simulink model "SFunctionModel"  (R2023b)
settings: Solver=VariableStepAuto  StartTime=0.0  StopTime=10.0  RelTol=1e-3
libraries: autolibshared x1
settings Model: Creator=Lenovo  LastModifiedBy=Lenovo

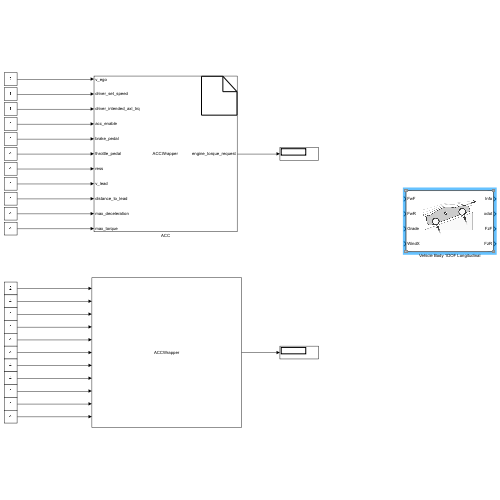
[thumbnail: Simulink's stored preview of the top-level diagram]
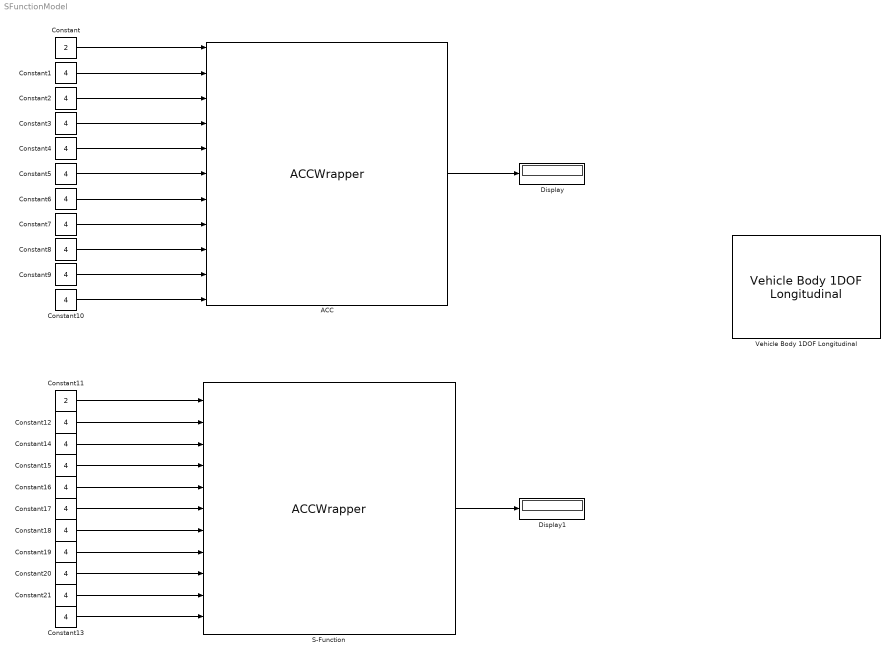
== system SFunctionModel ==
  ACC : S-Function  FunctionName=ACCWrapper  Parameters=1,4,1,1,1,1,1,1,1,1,1  SFunctionModules=ACCWrapper_wrapper.cpp  SFunctionDeploymentMode=off  EnableBusSupport=off  mask(S-Function Builder){}
      mask help: Simulink:masks:SFunctionBuilder_MD
      mask init:
      | val = [[.9  0.75 0.75 1 1 .9 .9 1]',[1 1 0.75 0.75 .9 .9 1 .9]'];try , sys = get_param(gcb,'SfunBuilderFcnName');if isempty(sys), sys = get_param(gcb,'FunctionName'); end,catch, sys = get_param(gcb,'FunctionName'); end
      settings: CopyFcn=set_param(gcbh,'LinkStatus','none')  OpenFcn=sfunctionwizard(gcbh)
      mask Display:
      | plot(val(:,1),val(:,2))
      | disp(sys)
      | port_label('input',1,'v_ego')
      | port_label('input',2,'driver_set_speed')
      | port_label('input',3,'driver_intended_axl_trq')
      | port_label('input',4,'acc_enable')
      | port_label('input',5,'brake_pedal')
      | port_label('input',6,'throttle_pedal')
      | port_label('input',7,'ress')
      | port_label('input',8,'v_lead')
      | port_label('input',9,'distance_to_lead')
      | port_label('input',10,'max_deceleration')
      | port_label('input',11,'max_torque')
      | port_label('output',1,'engine_torque_request')
  Constant : Constant  Value=2
  Constant{1..10,12..21} (20 alike) : Constant  Value=4
  Constant11 : Constant  Value=2
  Display : Display
  Display1 : Display
  S-Function : S-Function  FunctionName=ACCWrapper  Parameters=1,4,1,1,1,1,1,1,1,1,1  SFunctionModules=ACCWrapper.cpp  SFunctionDeploymentMode=off  EnableBusSupport=off
  Vehicle Body 1DOF Longitudinal : autolibshared/Vehicle Body 1DOF Longitudinal  VariantControl=SL  extFMode=off  extMMode=off  extTamb=off  wind3D=off  aMode=1  NF=2  NR=2  m=1500  a=1.4  b=1.8  h=.35  Cd=.3  Cl=0  Cpm=0  Af=4  x_o=0  xdot_o=0  Pabs=101325  T=273  g=9.81
      settings: LibrarySourceBlock=autolibvehdynlong/Vehicle Body 1DOF Longitudinal
  wires:
  Constant/1 -> ACC/1
  Constant1/1 -> ACC/2
  ACC/1 -> Display/1
  Constant2/1 -> ACC/3
  Constant3/1 -> ACC/4
  Constant4/1 -> ACC/5
  Constant5/1 -> ACC/6
  Constant6/1 -> ACC/7
  Constant7/1 -> ACC/8
  Constant8/1 -> ACC/9
  Constant9/1 -> ACC/10
  Constant10/1 -> ACC/11
  Constant11/1 -> S-Function/1
  Constant12/1 -> S-Function/2
  Constant14/1 -> S-Function/3
  Constant15/1 -> S-Function/4
  Constant16/1 -> S-Function/5
  Constant17/1 -> S-Function/6
  Constant18/1 -> S-Function/7
  Constant19/1 -> S-Function/8
  Constant20/1 -> S-Function/9
  Constant21/1 -> S-Function/10
  Constant13/1 -> S-Function/11
  S-Function/1 -> Display1/1
